simulink model "heading_control_models"  (R2017b)
settings: Solver=ode45  StartTime=tstart  StopTime=tstop  RelTol=1e-3  EnableMultiTasking=on
values from neighbouring files (symbols this model uses):
  c = 0    [TTK4190_A3_task1_2.m]    (also in TTK4190_A3_task1_3.m = 1; model_analysis.m; msfartoystyring.m = sqrt(cun*ur*n + cnn*n^2); sysID.m)
  dc = 3*deg2rad    (= 0.0523598775598)    [TTK4190_A3_task1_2.m]    (also in model_analysis.m = dc_list(i); sim_nomoto2.m = delta_c; sysID.m = dc_list(i))
  denum = 3.237*10^(-5)    (= 3.237e-05)    [TTK4190_A3_task1_3.m]    (also in parameters_heading_controller.m = 2.158e-05; sysID.m = 2.158e-05)
  denum_s = 0.009606    [TTK4190_A3_task1_3.m]    (also in parameters_heading_controller.m = 0.006835; sysID.m = 0.006835)
  K1 = 0.00466/dc    (= 0.088999444177)    [TTK4190_A3_task1_2.m]    (also in TTK4190_A3_task1_3.m = 0.089; parameters_heading_controller.m = 0.089)
  K2 = 0.00466/dc    (= 0.088999444177)    [TTK4190_A3_task1_2.m]    (also in TTK4190_A3_task1_3.m = -0.04)
  nc = 7.3    [TTK4190_A3_task1_2.m]    (also in TTK4190_A3_task1_3.m; model_analysis.m; parameters_heading_controller.m; sysID.m)
  num = -1.294*10^(-6)    (= -1.294e-06)    [TTK4190_A3_task1_3.m]    (also in parameters_heading_controller.m = -1.921e-06; sysID.m = -1.921e-06)
  num_s = -0.0003793    [TTK4190_A3_task1_3.m]    (also in parameters_heading_controller.m = -0.0003433; sysID.m = -0.0003433)
  p0 = zeros(2,1)    [TTK4190_A3_task1_2.m]    (also in TTK4190_A3_task1_3.m; model_analysis.m; sysID.m)
  psi0 = 0    [TTK4190_A3_task1_2.m]    (also in TTK4190_A3_task1_3.m; model_analysis.m; sysID.m)
  r0 = 0    [TTK4190_A3_task1_2.m]    (also in TTK4190_A3_task1_3.m; model_analysis.m; sysID.m)
  T = 197.5    [TTK4190_A3_task1_2.m]    (also in TTK4190_A3_task1_3.m; model_analysis.m = x(1); parameters_heading_controller.m)
  T1 = 250    [TTK4190_A3_task1_2.m]    (also in TTK4190_A3_task1_3.m = 204; model_analysis.m = x(1))
  T2 = 325    [TTK4190_A3_task1_2.m]    (also in TTK4190_A3_task1_3.m = 224; model_analysis.m = x(2))
  T3 = 490    [TTK4190_A3_task1_2.m]    (also in TTK4190_A3_task1_3.m = 423; model_analysis.m = x(3))
  tsamp = 10    [TTK4190_A3_task1_2.m]    (also in TTK4190_A3_task1_3.m; model_analysis.m = 35; sim_nomoto2.m = tsamp; sysID.m = 100)
  v0 = [6.63 0]'    [TTK4190_A3_task1_2.m]    (also in TTK4190_A3_task1_3.m; model_analysis.m; sysID.m)
undefined symbols (not defined in the file or in its folder): msfartoystyring
settings Model: ExtModeAutoUpdateStatusClock=off  Creator=christh  LastModifiedBy=Marie
settings DataIOCC: LimitDataPoints=on  SaveFormat=Array  SignalLoggingSaveFormat=ModelDataLogs
settings OptimizationCC: ExpressionDepthLimit=2147483647  InitFltsAndDblsToZero=on  LifeSpan=inf
settings DebuggingCC: UnderspecifiedInitializationDetection=Classic  MergeDetectMultiDrivingBlocksExec=none  SolverPrmCheckMsg=warning  FcnCallInpInsideContextMsg=warning  StateNameClashWarn=warning  SFUnexpectedBacktrackingDiag=warning  SFNoUnconditionalDefaultTransitionDiag=warning  SFExecutionAtInitializationDiag=none
settings HardwareCC: ProdBitPerPointer=32  ProdBitPerSizeT=32  ProdBitPerPtrDiffT=32  ProdLargestAtomicFloat=None  ProdIntDivRoundTo=Undefined  ProdEndianess=Unspecified  ProdWordSize=32  ProdHWDeviceType=32-bit Generic
settings ModelReferenceCC: PropagateSignalLabelsOutOfModel=off
settings CodeAppCC: StateflowObjectComments=on
settings GRTTargetCC: TargetLangStandard=C89/C90 (ANSI)  GeneratePreprocessorConditionals=Disable all  CombineOutputUpdateFcns=off  GRTInterface=on
settings ConfigComp: CovMetricSettings=dw  CovHtmlReporting=on  CovSaveCumulativeToWorkspaceVar=on  CovSaveSingleToWorkspaceVar=on  CovExternalEMLEnable=off

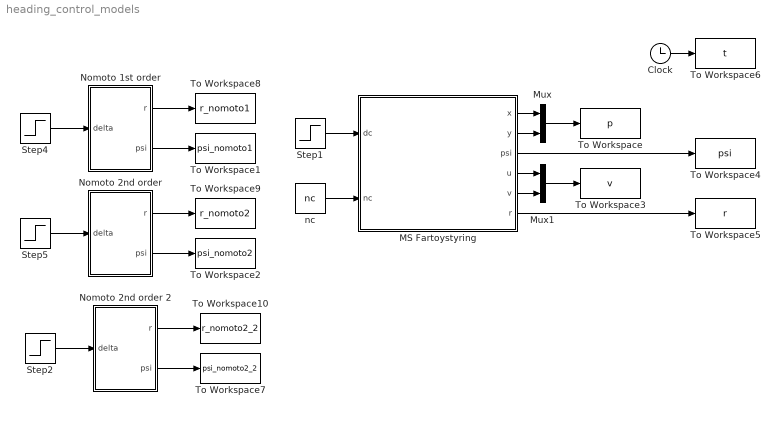
== system heading_control_models ==
  Clock : Clock
  MS Fartoystyring : Subsystem  mask(MS Fartoystyring for Assignment 3 G&C){x0=p0(1), y0=p0(2), u0=v0(1), v0=v0(2), psi0=psi0, r0=r0, c=c}
      mask prompts: x0 "x(t0) (m)"; y0 "y(t0) (m)"; u0 "u(t0) (m/s)"; v0 "v(t0) (m/s)"; psi0 "psi(t0) (rad)"; r0 "r(t0) (rad/s)"; c "current (0 or 1)"
      mask help:
      | Block corresponding to Figure 1 in the assignment text. Gives the response of the ship.
      |
      | The design speed of MS Fartoystyring is u=8.23 m/s.
      |
      | Input:
      | dc: commanded rudder (rad), dmax=25*pi/180
      | nc: commanded shaft speed (rad/s), nmax=85*2*pi/60
      |
      | Output:
      | x: north pos (m)
      | y: east pos (m)
      | u: surge (m/s)
      | v: sway (m/s)
      | psi: heading (rad)
      | r: yaw (rad/s)
      mask Help: Comments, bugs and help requests can be directed to the TA. Email on course website.
  Mux : Mux  Inputs=2
  Mux1 : Mux  Inputs=2
  Nomoto 1st order : Subsystem
  Nomoto 2nd order : Subsystem
  Nomoto 2nd order 2 : Subsystem
  Step{1..2,4..5} (4 alike) : Step  After=dc  SampleTime=0
  To Workspace : ToWorkspace  VariableName=p  SampleTime=tsamp
  To Workspace1 : ToWorkspace  VariableName=psi_nomoto1  SampleTime=tsamp
  To Workspace10 : ToWorkspace  VariableName=r_nomoto2_2  SampleTime=tsamp
  To Workspace2 : ToWorkspace  VariableName=psi_nomoto2  SampleTime=tsamp
  To Workspace3 : ToWorkspace  VariableName=v  SampleTime=tsamp
  To Workspace4 : ToWorkspace  VariableName=psi  SampleTime=tsamp
  To Workspace5 : ToWorkspace  VariableName=r  SampleTime=tsamp
  To Workspace6 : ToWorkspace  VariableName=t  SampleTime=tsamp
  To Workspace7 : ToWorkspace  VariableName=psi_nomoto2_2  SampleTime=tsamp
  To Workspace8 : ToWorkspace  VariableName=r_nomoto1  SampleTime=tsamp
  To Workspace9 : ToWorkspace  VariableName=r_nomoto2  SampleTime=tsamp
  nc : Constant  Value=nc
  wires:
  Clock/1 -> To Workspace6/1
  MS Fartoystyring/1(x) -> Mux/1
  MS Fartoystyring/2(y) -> Mux/2
  MS Fartoystyring/4(u) -> Mux1/1
  MS Fartoystyring/5(v) -> Mux1/2
  Mux/1 -> To Workspace/1
  Mux1/1 -> To Workspace3/1
  MS Fartoystyring/3(psi) -> To Workspace4/1
  MS Fartoystyring/6(r) -> To Workspace5/1
  nc/1 -> MS Fartoystyring/2(nc)
  Step1/1 -> MS Fartoystyring/1(dc)
  Nomoto 1st order/1(r) -> To Workspace8/1
  Step4/1 -> Nomoto 1st order/1(delta)
  Step5/1 -> Nomoto 2nd order/1(delta)
  Nomoto 2nd order/1(r) -> To Workspace9/1
  Nomoto 1st order/2(psi) -> To Workspace1/1
  Nomoto 2nd order/2(psi) -> To Workspace2/1
  Nomoto 2nd order 2/1(r) -> To Workspace10/1
  Nomoto 2nd order 2/2(psi) -> To Workspace7/1
  Step2/1 -> Nomoto 2nd order 2/1(delta)

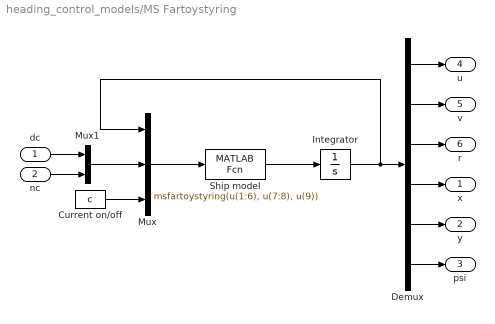
== system heading_control_models/MS Fartoystyring ==
  dc : Inport
  nc : Inport  Port=2
  Current on/off : Constant  Value=c
  Demux : Demux  Outputs=6
  Integrator : Integrator  InitialCondition=[u0 v0 r0 x0 y0 psi0]'
  Mux : Mux  Inputs=3
  Mux1 : Mux  Inputs=2
  Ship model : MATLABFcn  MATLABFcn=msfartoystyring(u(1:6), u(7:8), u(9))  OutputDimensions=6
  x : Outport
  y : Outport  Port=2
  psi : Outport  Port=3
  u : Outport  Port=4
  v : Outport  Port=5
  r : Outport  Port=6
  wires:
  Integrator/1 -> Mux/1, Demux/1
  Mux1/1 -> Mux/2
  dc/1 -> Mux1/1
  nc/1 -> Mux1/2
  Demux/1 -> u/1
  Demux/2 -> v/1
  Demux/3 -> r/1
  Demux/4 -> x/1
  Demux/5 -> y/1
  Demux/6 -> psi/1
  Current on/off/1 -> Mux/3
  Ship model/1 -> Integrator/1
  Mux/1 -> Ship model/1

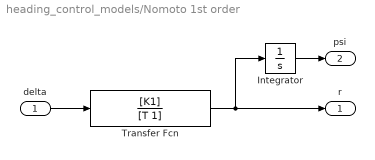
== system heading_control_models/Nomoto 1st order ==
  delta : Inport
  Integrator : Integrator
  Transfer Fcn : TransferFcn  Numerator=[K1]  Denominator=[T 1]
  r : Outport
  psi : Outport  Port=2
  wires:
  delta/1 -> Transfer Fcn/1
  Integrator/1 -> psi/1
  Transfer Fcn/1 -> Integrator/1, r/1

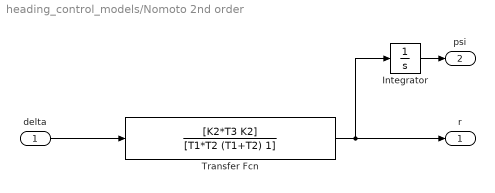
== system heading_control_models/Nomoto 2nd order ==
  delta : Inport
  Integrator : Integrator
  Transfer Fcn : TransferFcn  Numerator=[K2*T3 K2]  Denominator=[T1*T2 (T1+T2) 1]
  r : Outport
  psi : Outport  Port=2
  wires:
  delta/1 -> Transfer Fcn/1
  Integrator/1 -> psi/1
  Transfer Fcn/1 -> Integrator/1, r/1

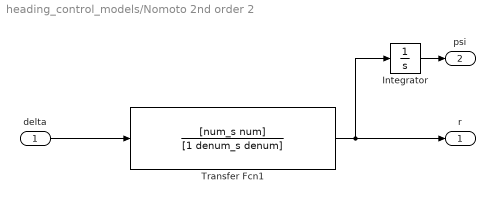
== system heading_control_models/Nomoto 2nd order 2 ==
  delta : Inport
  Integrator : Integrator
  Transfer Fcn1 : TransferFcn  Numerator=[num_s num]  Denominator=[1 denum_s denum]
  r : Outport
  psi : Outport  Port=2
  wires:
  delta/1 -> Transfer Fcn1/1
  Integrator/1 -> psi/1
  Transfer Fcn1/1 -> Integrator/1, r/1
